simulink model "three_way_newest_1"  (R2025b)
settings: Solver=VariableStepAuto  StartTime=0.0  StopTime=20  RelTol=1e-3
undefined symbols (not defined in the file or in its folder): c, dspblkCoreblockFVToolHelper, gcbh, sfvc784, xck26
libraries: hdlBasic x131, hdlDSPIP x11, simulink x10, hdlUtilities x4, vmcUtilities x1
(part 1 of 2)
settings Model: Creator=janek  LastModifiedBy=janek

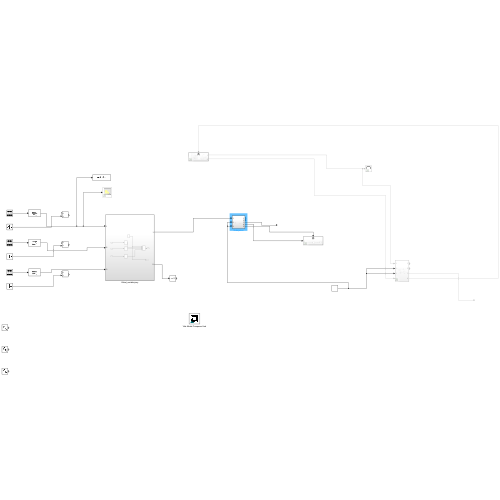
[thumbnail: Simulink's stored preview of the top-level diagram]
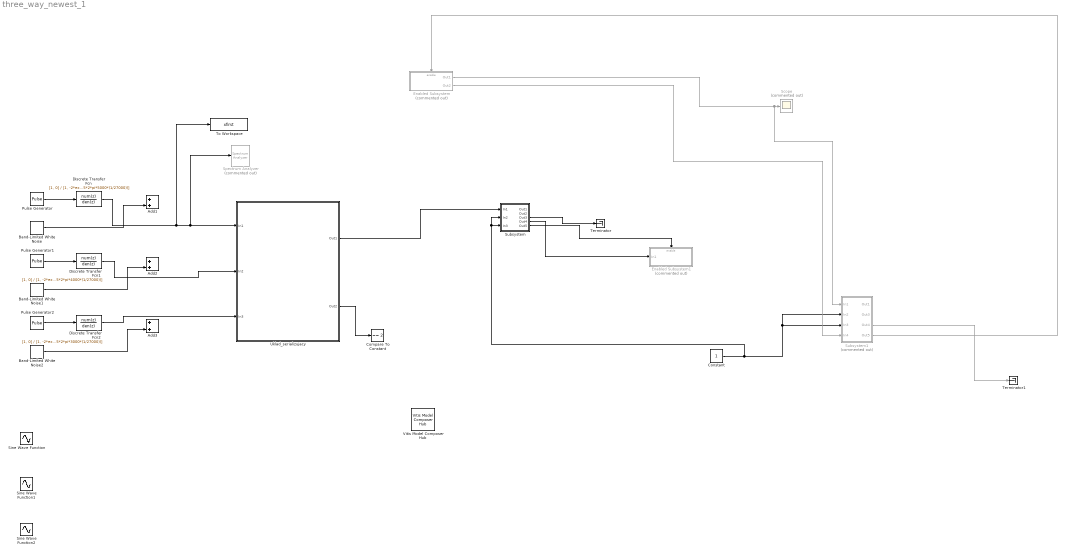
== system three_way_newest_1 ==
  Add1 : Sum
  Add2 : Sum
  Add3 : Sum
  Band-Limited White Noise : simulink/Sources/Band-Limited White Noise  Cov=[0.000001]  Ts=1/27000  seed=[23341]
  Band-Limited White Noise1 : simulink/Sources/Band-Limited White Noise  Cov=[0.000005]  Ts=1/27000  seed=[23341]
  Band-Limited White Noise2 : simulink/Sources/Band-Limited White Noise  Cov=[0.000005]  Ts=1/27000  seed=[23341]
  Compare To Constant : simulink/Logic and Bit Operations/Compare To Constant  relop===  const=2  OutDataTypeStr=boolean
  Constant : Constant
  Discrete Transfer Fcn : DiscreteTransferFcn  LoadFcn=dspblkCoreblockFVToolHelper(gcbh,'load');  Numerator=[1, 0]  Denominator=[1, -2*exp(-0.05*2*pi*5000*(1/27000))*cos(2*pi*5000*sqrt(1-0.05^2)*(1/27000)), exp(-2*0.05*2*pi*5000*(1/27000))]
      settings: CopyFcn=dspblkCoreblockFVToolHelper(gcbh,'copy');  DeleteFcn=dspblkCoreblockFVToolHelper(gcbh,'close');  ModelCloseFcn=dspblkCoreblockFVToolHelper(gcbh,'close');  PreSaveFcn=dspblkCoreblockFVToolHelper(gcbh,'presave');  PostSaveFcn=dspblkCoreblockFVToolHelper(gcbh,'postsave');  CloseFcn=dspblkCoreblockFVToolHelper(gcbh,'close');
  Discrete Transfer Fcn1 : DiscreteTransferFcn  LoadFcn=dspblkCoreblockFVToolHelper(gcbh,'load');  Numerator=[1, 0]  Denominator=[1, -2*exp(-0.05*2*pi*5000*(1/27000))*cos(2*pi*4000*sqrt(1-0.05^2)*(1/27000)), exp(-2*0.05*2*pi*4000*(1/27000))]
      settings: CopyFcn=dspblkCoreblockFVToolHelper(gcbh,'copy');  DeleteFcn=dspblkCoreblockFVToolHelper(gcbh,'close');  ModelCloseFcn=dspblkCoreblockFVToolHelper(gcbh,'close');  PreSaveFcn=dspblkCoreblockFVToolHelper(gcbh,'presave');  PostSaveFcn=dspblkCoreblockFVToolHelper(gcbh,'postsave');  CloseFcn=dspblkCoreblockFVToolHelper(gcbh,'close');
  Discrete Transfer Fcn2 : DiscreteTransferFcn  LoadFcn=dspblkCoreblockFVToolHelper(gcbh,'load');  Numerator=[1, 0]  Denominator=[1, -2*exp(-0.05*2*pi*5000*(1/27000))*cos(2*pi*3000*sqrt(1-0.05^2)*(1/27000)), exp(-2*0.05*2*pi*3000*(1/27000))]
      settings: CopyFcn=dspblkCoreblockFVToolHelper(gcbh,'copy');  DeleteFcn=dspblkCoreblockFVToolHelper(gcbh,'close');  ModelCloseFcn=dspblkCoreblockFVToolHelper(gcbh,'close');  PreSaveFcn=dspblkCoreblockFVToolHelper(gcbh,'presave');  PostSaveFcn=dspblkCoreblockFVToolHelper(gcbh,'postsave');  CloseFcn=dspblkCoreblockFVToolHelper(gcbh,'close');
  Enabled Subsystem : Subsystem  Commented=on  TreatAsAtomicUnit=on
  Enabled Subsystem1 : Subsystem  Commented=on  TreatAsAtomicUnit=on
  Pulse Generator : DiscretePulseGenerator  Period=540  SampleTime=1/27000
  Pulse Generator1 : DiscretePulseGenerator  Period=675  SampleTime=1/27000
  Pulse Generator2 : DiscretePulseGenerator  Period=900  SampleTime=1/27000
  Scope : Scope  Commented=on
      settings: ActiveDisplayYMinimum=-1.152524294390888  ActiveDisplayYMaximum=1.239169366043442  DataLoggingVariableName=ScopeData15
  Sine Wave Function : Sin  Frequency=2*pi*4000  SampleTime=1/27000
  Sine Wave Function1 : Sin  Frequency=2*pi*5000  SampleTime=1/27000
  Sine Wave Function2 : Sin  Frequency=2*pi*3000  SampleTime=1/27000
  Spectrum Analyzer : SpectrumAnalyzer  Commented=on  WindowPosition=[993.000000,73.000000,800.000000,500.000000,]  ScopeFrameLocation=window  WindowInvariantSamplesPerUpdate=on  Span=27000  StartFrequency=-13500  StopFrequency=13500  YLimits=[-53.93 -0.0586]  SelectedToolstripTab=spectrumAnalyzerToolstrip.measurementsTab
  Subsystem : Subsystem
  Subsystem1 : Subsystem  Commented=on
  Terminator : Terminator
  Terminator1 : Terminator
  To Workspace : ToWorkspace  VariableName=xfirst  SampleTime=-1
  Uklad_serializujacy : Subsystem
  Vitis Model Composer Hub : vmcUtilities/Vitis Model Composer Hub  Tag=genX  CodeGeneration=off  SubsystemName=Subsystem  CompilationType=HDLCompilation  ExportTypeV2=IP Catalog  StartColumn=1  NumberOfColumns=1  TargetDirectory=./netlist  exportDesign=off  analyzeDesign=off  validateDesignOnHw=off  ExportType=AI Engines  IpVendor=xilinx.com  IpLibrary=hls  IpVersion=1.0  IpHWLanguage=Verilog  AieCompilerOptions={}  AieSimulatorOptions={}  CreateTestbench=off  TestbenchStackSize=10  RunRtlSim=off  RunCSim=off  RunAieSim=off  AieSimTimeout=50000  RunAieSimProfiling=off  LaunchVitisAnalyzer=off  PlotOutput=off  RunX86Sim=off  X86SimTimeout=10  GenHwImage=off  GenLibadfXo=on  GenHwValidationCode=off  PlatformType=Not Specified  HwSystemType=Baremetal  HwValidationTarget=hw  ProjDevice=Kria KR260 Robotics Starter Kit SOM (xck26-sfvc784-2LV-c)  ProjDevicePart=xck26-sfvc784-2LV-c  AIEType=None  SamplePeriod=-1  ClockFrequency=200  DataPathParallelism=1  xilinxfamily=zynquplus  part=xck26  speed=-2LV-c  package=sfvc784  directory=./netlist\ip\Subsystem\src  testbench=off  incr_netlist=off  synthesis_tool=Vivado  clock_wrapper=Clock Enables  dbl_ovrd=According to Block Masks  dcm_input_clock_period=10  sysclk_period=1000  simulink_period=1/81000  eval_field=0  LogFileName=''  NThreads=4
  wires:
  Discrete Transfer Fcn/1 -> To Workspace/1, Spectrum Analyzer/1, Uklad_serializujacy/1(In1)
  Band-Limited White Noise/1 -> Add1/2
  Discrete Transfer Fcn1/1 -> Uklad_serializujacy/2(In2)
  Pulse Generator1/1 -> Discrete Transfer Fcn1/1
  Band-Limited White Noise1/1 -> Add2/2
  Discrete Transfer Fcn2/1 -> Uklad_serializujacy/3(In3)
  Subsystem1/3(Out4) -> Terminator1/1
  Pulse Generator/1 -> Discrete Transfer Fcn/1
  Constant/1 -> Subsystem/3(In3), Subsystem/2(In2), Subsystem1/2(In2), Subsystem1/3(In3)
  Band-Limited White Noise2/1 -> Add3/2
  Pulse Generator2/1 -> Discrete Transfer Fcn2/1
  Uklad_serializujacy/2(Out2) -> Compare To Constant/1
  Enabled Subsystem/2(Out2) -> Subsystem1/4(In4)
  Enabled Subsystem/1(Out1) -> Scope/1, Subsystem1/1(In1)
  Subsystem1/4(Out5) -> Enabled Subsystem/Enable
  Subsystem/3(Out3) -> Terminator/1
  Uklad_serializujacy/1(Out1) -> Subsystem/1(In1)
  Subsystem/4(Out4) -> Enabled Subsystem1/1(In1)
  Subsystem/5(Out5) -> Enabled Subsystem1/Enable

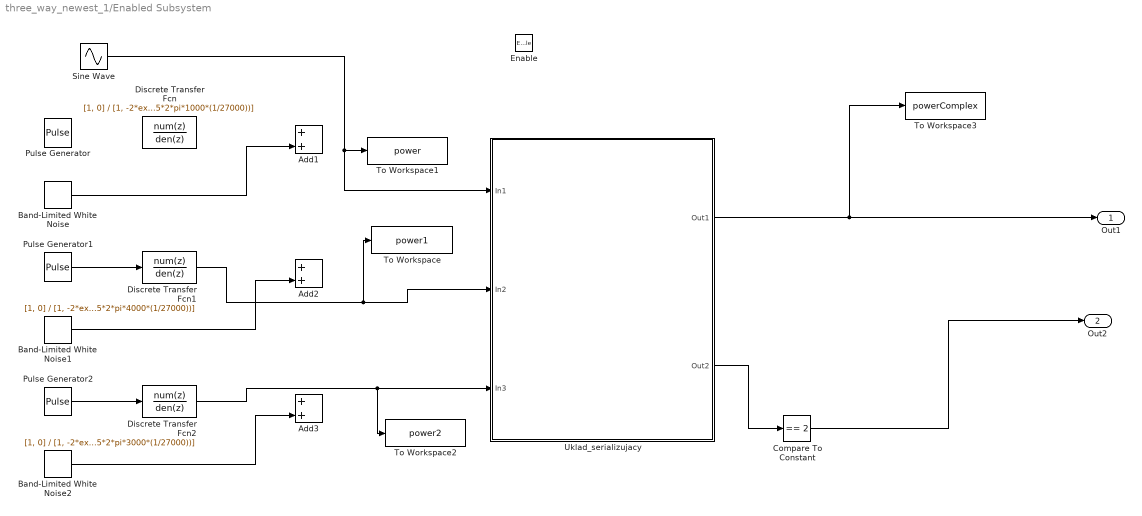
== system three_way_newest_1/Enabled Subsystem ==
  Enable : EnablePort
  Add1 : Sum
  Add2 : Sum
  Add3 : Sum
  Band-Limited White Noise : simulink/Sources/Band-Limited White Noise  Cov=[0.000001]  Ts=1/27000  seed=[23341]
  Band-Limited White Noise1 : simulink/Sources/Band-Limited White Noise  Cov=[0.000005]  Ts=1/27000  seed=[23341]
  Band-Limited White Noise2 : simulink/Sources/Band-Limited White Noise  Cov=[0.000005]  Ts=1/27000  seed=[23341]
  Compare To Constant : simulink/Logic and Bit Operations/Compare To Constant  relop===  const=2  OutDataTypeStr=boolean
  Discrete Transfer Fcn : DiscreteTransferFcn  LoadFcn=dspblkCoreblockFVToolHelper(gcbh,'load');  Numerator=[1, 0]  Denominator=[1, -2*exp(-0.05*2*pi*5000*(1/27000))*cos(2*pi*1000*sqrt(1-0.05^2)*(1/27000)), exp(-2*0.05*2*pi*1000*(1/27000))]
      settings: CopyFcn=dspblkCoreblockFVToolHelper(gcbh,'copy');  DeleteFcn=dspblkCoreblockFVToolHelper(gcbh,'close');  ModelCloseFcn=dspblkCoreblockFVToolHelper(gcbh,'close');  PreSaveFcn=dspblkCoreblockFVToolHelper(gcbh,'presave');  PostSaveFcn=dspblkCoreblockFVToolHelper(gcbh,'postsave');  CloseFcn=dspblkCoreblockFVToolHelper(gcbh,'close');
  Discrete Transfer Fcn1 : DiscreteTransferFcn  LoadFcn=dspblkCoreblockFVToolHelper(gcbh,'load');  Numerator=[1, 0]  Denominator=[1, -2*exp(-0.05*2*pi*5000*(1/27000))*cos(2*pi*4000*sqrt(1-0.05^2)*(1/27000)), exp(-2*0.05*2*pi*4000*(1/27000))]
      settings: CopyFcn=dspblkCoreblockFVToolHelper(gcbh,'copy');  DeleteFcn=dspblkCoreblockFVToolHelper(gcbh,'close');  ModelCloseFcn=dspblkCoreblockFVToolHelper(gcbh,'close');  PreSaveFcn=dspblkCoreblockFVToolHelper(gcbh,'presave');  PostSaveFcn=dspblkCoreblockFVToolHelper(gcbh,'postsave');  CloseFcn=dspblkCoreblockFVToolHelper(gcbh,'close');
  Discrete Transfer Fcn2 : DiscreteTransferFcn  LoadFcn=dspblkCoreblockFVToolHelper(gcbh,'load');  Numerator=[1, 0]  Denominator=[1, -2*exp(-0.05*2*pi*5000*(1/27000))*cos(2*pi*3000*sqrt(1-0.05^2)*(1/27000)), exp(-2*0.05*2*pi*3000*(1/27000))]
      settings: CopyFcn=dspblkCoreblockFVToolHelper(gcbh,'copy');  DeleteFcn=dspblkCoreblockFVToolHelper(gcbh,'close');  ModelCloseFcn=dspblkCoreblockFVToolHelper(gcbh,'close');  PreSaveFcn=dspblkCoreblockFVToolHelper(gcbh,'presave');  PostSaveFcn=dspblkCoreblockFVToolHelper(gcbh,'postsave');  CloseFcn=dspblkCoreblockFVToolHelper(gcbh,'close');
  Pulse Generator : DiscretePulseGenerator  Period=540  SampleTime=1/27000
  Pulse Generator1 : DiscretePulseGenerator  Period=675  SampleTime=1/27000
  Pulse Generator2 : DiscretePulseGenerator  Period=900  SampleTime=1/27000
  Sine Wave : Sin  Frequency=2*pi*1000  SampleTime=1/27000
  To Workspace : ToWorkspace  VariableName=power1  SampleTime=-1
  To Workspace1 : ToWorkspace  VariableName=power  SampleTime=-1
  To Workspace2 : ToWorkspace  VariableName=power2  SampleTime=-1
  To Workspace3 : ToWorkspace  VariableName=powerComplex  SampleTime=-1
  Uklad_serializujacy : Subsystem
  Out1 : Outport
  Out2 : Outport  Port=2
  wires:
  Band-Limited White Noise/1 -> Add1/2
  Pulse Generator2/1 -> Discrete Transfer Fcn2/1
  Discrete Transfer Fcn1/1 -> To Workspace/1, Uklad_serializujacy/2(In2)
  Discrete Transfer Fcn2/1 -> To Workspace2/1, Uklad_serializujacy/3(In3)
  Band-Limited White Noise1/1 -> Add2/2
  Uklad_serializujacy/2(Out2) -> Compare To Constant/1
  Band-Limited White Noise2/1 -> Add3/2
  Pulse Generator1/1 -> Discrete Transfer Fcn1/1
  Uklad_serializujacy/1(Out1) -> To Workspace3/1, Out1/1
  Compare To Constant/1 -> Out2/1
  Sine Wave/1 -> Uklad_serializujacy/1(In1), To Workspace1/1

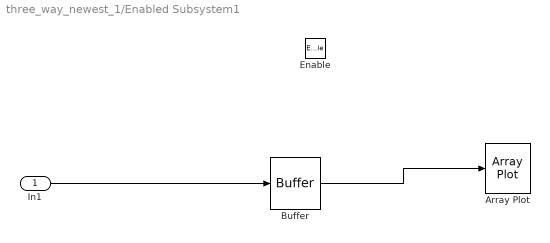
== system three_way_newest_1/Enabled Subsystem1 ==
  In1 : Inport
  Enable : EnablePort
  Array Plot : ArrayPlot  WindowPosition=[372.000000,68.000000,800.000000,500.000000,]  ScopeFrameLocation=window  YLimits=[0.875 1.125]
  Buffer : Buffer  N=4096  OutputFrames=off
  wires:
  In1/1 -> Buffer/1
  Buffer/1 -> Array Plot/1

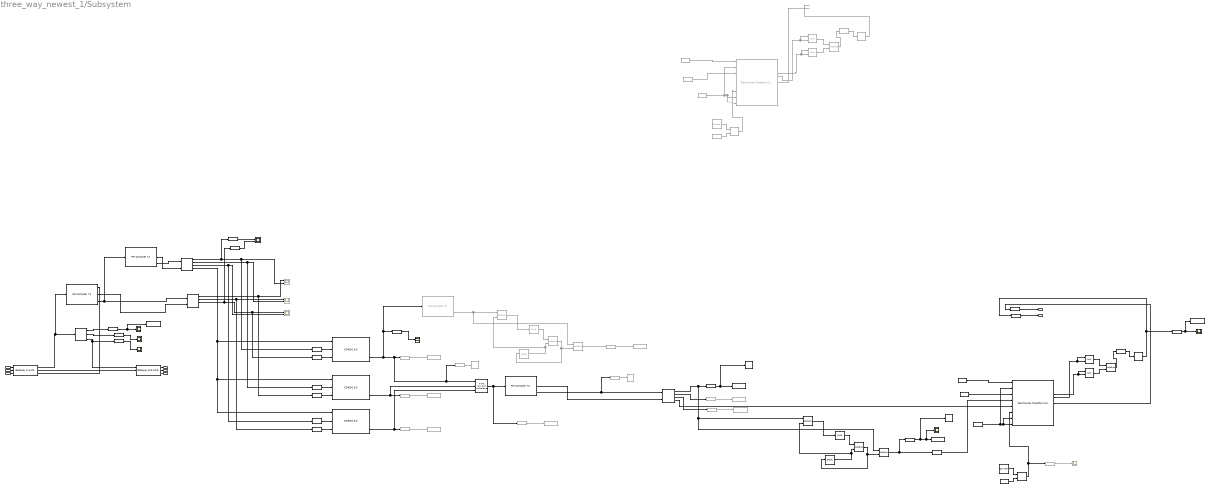
== system three_way_newest_1/Subsystem ==
  In1 : Inport
  In2 : Inport  Port=2
  In3 : Inport  Port=3
  AddSub : hdlBasic/AddSub  Commented=on  mode=Addition  use_carryin=off  use_carryout=off  en=off  latency=0  precision=User Defined  arith_type="Signed  (2's comp)"  n_bits=32  bin_pt=26  quantization="Round  (unbiased: +/- Inf)"  overflow=Wrap  use_behavioral_HDL=off  hw_selection=Fabric  pipelined=off  XmcBlockStatus=1  maskContainerNames=tabcontainer1  block_type=addsub  block_config=sysgen:Addsub_config
  AddSub1 : hdlBasic/AddSub  Commented=on  mode=Subtraction  use_carryin=off  use_carryout=off  en=off  latency=0  precision=User Defined  arith_type="Signed  (2's comp)"  n_bits=32  bin_pt=26  quantization="Round  (unbiased: +/- Inf)"  overflow=Wrap  use_behavioral_HDL=off  hw_selection=Fabric  pipelined=off  XmcBlockStatus=1  maskContainerNames=tabcontainer1  block_type=addsub  block_config=sysgen:Addsub_config
  AddSub2 : hdlBasic/AddSub  Commented=on  mode=Subtraction  use_carryin=off  use_carryout=off  en=off  latency=0  precision=User Defined  arith_type="Signed  (2's comp)"  n_bits=16  bin_pt=12  quantization="Round  (unbiased: +/- Inf)"  overflow=Saturate  use_behavioral_HDL=off  hw_selection=Fabric  pipelined=off  XmcBlockStatus=1  maskContainerNames=tabcontainer1  block_type=addsub  block_config=sysgen:Addsub_config
  AddSub3 : hdlBasic/AddSub  mode=Addition  use_carryin=off  use_carryout=off  en=off  latency=0  precision=Full  arith_type=Unsigned  n_bits=16  bin_pt=14  quantization=Truncate  overflow=Wrap  use_behavioral_HDL=off  hw_selection=Fabric  pipelined=off  XmcBlockStatus=1  maskContainerNames=tabcontainer1  block_type=addsub  block_config=sysgen:Addsub_config
  AddSub4 : hdlBasic/AddSub  Commented=on  mode=Addition  use_carryin=off  use_carryout=off  en=off  latency=0  precision=Full  arith_type=Unsigned  n_bits=16  bin_pt=14  quantization=Truncate  overflow=Wrap  use_behavioral_HDL=off  hw_selection=Fabric  pipelined=off  XmcBlockStatus=1  maskContainerNames=tabcontainer1  block_type=addsub  block_config=sysgen:Addsub_config
  AddSub5 : hdlBasic/AddSub  mode=Addition  use_carryin=off  use_carryout=off  en=off  latency=0  precision=User Defined  arith_type="Signed  (2's comp)"  n_bits=32  bin_pt=26  quantization="Round  (unbiased: +/- Inf)"  overflow=Wrap  use_behavioral_HDL=off  hw_selection=Fabric  pipelined=off  XmcBlockStatus=1  maskContainerNames=tabcontainer1  block_type=addsub  block_config=sysgen:Addsub_config
  AddSub6 : hdlBasic/AddSub  mode=Subtraction  use_carryin=off  use_carryout=off  en=off  latency=0  precision=User Defined  arith_type="Signed  (2's comp)"  n_bits=32  bin_pt=26  quantization="Round  (unbiased: +/- Inf)"  overflow=Wrap  use_behavioral_HDL=off  hw_selection=Fabric  pipelined=off  XmcBlockStatus=1  maskContainerNames=tabcontainer1  block_type=addsub  block_config=sysgen:Addsub_config
  AddSub7 : hdlBasic/AddSub  mode=Subtraction  use_carryin=off  use_carryout=off  en=off  latency=0  precision=User Defined  arith_type="Signed  (2's comp)"  n_bits=16  bin_pt=12  quantization="Round  (unbiased: +/- Inf)"  overflow=Saturate  use_behavioral_HDL=off  hw_selection=Fabric  pipelined=off  XmcBlockStatus=1  maskContainerNames=tabcontainer1  block_type=addsub  block_config=sysgen:Addsub_config
  "CORDIC 6.0 " : hdlDSPIP/CORDIC 6.0   functional_selection=Translate  architectural_configuration=Parallel  pipelining_mode=Maximum  data_format=SignedFraction  phase_format=Radians  input_width=16  output_width=16  round_mode=Nearest_Even  iterations=0  precision=0  compensation_scaling=BRAM  coarse_rotation=on  aclken=off  aresetn=off  out_tready=off  cartesian_has_tuser=off  cartesian_has_tlast=off  cartesian_tuser_width=1  phase_has_tuser=off  phase_has_tlast=off  phase_tuser_width=1  out_tlast_behv=Null  flow_control=NonBlocking  optimize_goal=Resources  trim_axipin_name=on  simulation_type=hybrid_sim  simulation_model=sysgen:cordic_v6_0  data_path_portlist={'s_axis_cartesian_tdata_imag', 's_axis_cartesian_tdata_real', 's_axis_phase_tdata_phase', 'm_axis_dout_tdata_imag', 'm_axis_dout_tdata_real', 'm_axis_dout_tdata_phase','m_axis_dout_tdata'}  ip_name=CORDIC  ip_version=6.0  dsptool_ready=true  ipcore_usecache=true  ipcore_useipmodelcache=true  wrapper_available=true  port_translation_map={ 'aclken' => 'en', 'aresetn' => 'rst' }  XmcBlockStatus=1  maskContainerNames=group15  block_type=cordic_v6_0  block_config=sysgen:rodinimport_config  block_width=800
  CORDIC 6.0 1 : hdlDSPIP/CORDIC 6.0   functional_selection=Translate  architectural_configuration=Parallel  pipelining_mode=Maximum  data_format=SignedFraction  phase_format=Radians  input_width=16  output_width=16  round_mode=Nearest_Even  iterations=0  precision=0  compensation_scaling=BRAM  coarse_rotation=on  aclken=off  aresetn=off  out_tready=off  cartesian_has_tuser=off  cartesian_has_tlast=off  cartesian_tuser_width=1  phase_has_tuser=off  phase_has_tlast=off  phase_tuser_width=1  out_tlast_behv=Null  flow_control=NonBlocking  optimize_goal=Resources  trim_axipin_name=on  simulation_type=hybrid_sim  simulation_model=sysgen:cordic_v6_0  data_path_portlist={'s_axis_cartesian_tdata_imag', 's_axis_cartesian_tdata_real', 's_axis_phase_tdata_phase', 'm_axis_dout_tdata_imag', 'm_axis_dout_tdata_real', 'm_axis_dout_tdata_phase','m_axis_dout_tdata'}  ip_name=CORDIC  ip_version=6.0  dsptool_ready=true  ipcore_usecache=true  ipcore_useipmodelcache=true  wrapper_available=true  port_translation_map={ 'aclken' => 'en', 'aresetn' => 'rst' }  XmcBlockStatus=1  maskContainerNames=group15  block_type=cordic_v6_0  block_config=sysgen:rodinimport_config  block_width=800
  CORDIC 6.0 2 : hdlDSPIP/CORDIC 6.0   functional_selection=Translate  architectural_configuration=Parallel  pipelining_mode=Maximum  data_format=SignedFraction  phase_format=Radians  input_width=16  output_width=16  round_mode=Nearest_Even  iterations=0  precision=0  compensation_scaling=BRAM  coarse_rotation=on  aclken=off  aresetn=off  out_tready=off  cartesian_has_tuser=off  cartesian_has_tlast=off  cartesian_tuser_width=1  phase_has_tuser=off  phase_has_tlast=off  phase_tuser_width=1  out_tlast_behv=Null  flow_control=NonBlocking  optimize_goal=Resources  trim_axipin_name=on  simulation_type=hybrid_sim  simulation_model=sysgen:cordic_v6_0  data_path_portlist={'s_axis_cartesian_tdata_imag', 's_axis_cartesian_tdata_real', 's_axis_phase_tdata_phase', 'm_axis_dout_tdata_imag', 'm_axis_dout_tdata_real', 'm_axis_dout_tdata_phase','m_axis_dout_tdata'}  ip_name=CORDIC  ip_version=6.0  dsptool_ready=true  ipcore_usecache=true  ipcore_useipmodelcache=true  wrapper_available=true  port_translation_map={ 'aclken' => 'en', 'aresetn' => 'rst' }  XmcBlockStatus=1  maskContainerNames=group15  block_type=cordic_v6_0  block_config=sysgen:rodinimport_config  block_width=800
  Constant : hdlBasic/Constant  Commented=on  const=0  gui_display_data_type=Fixed-point  arith_type=Signed (2's comp)  n_bits=16  bin_pt=15  preci_type=Single  exp_width=8  frac_width=24  explicit_period=off  period=1  XmcBlockStatus=1  maskContainerNames=tabcontainer1  block_type=constant  block_config=sysgen:Constant_config
  Constant1 : hdlBasic/Constant  Commented=on  const=1  gui_display_data_type=Boolean  arith_type=Boolean  n_bits=1  bin_pt=0  preci_type=Single  exp_width=8  frac_width=24  explicit_period=off  period=1  XmcBlockStatus=1  maskContainerNames=tabcontainer1  block_type=constant  block_config=sysgen:Constant_config
  Constant2 : hdlBasic/Constant  const=0  gui_display_data_type=Fixed-point  arith_type=Signed (2's comp)  n_bits=16  bin_pt=15  preci_type=Single  exp_width=8  frac_width=24  explicit_period=off  period=1  XmcBlockStatus=1  maskContainerNames=tabcontainer1  block_type=constant  block_config=sysgen:Constant_config
  Constant3 : hdlBasic/Constant  Commented=on  const=1  gui_display_data_type=Fixed-point  arith_type=Unsigned  n_bits=1  bin_pt=0  preci_type=Single  exp_width=8  frac_width=24  explicit_period=off  period=1  XmcBlockStatus=1  maskContainerNames=tabcontainer1  block_type=constant  block_config=sysgen:Constant_config
  Constant4 : hdlBasic/Constant  Commented=on  const=4095  gui_display_data_type=Fixed-point  arith_type=Unsigned  n_bits=12  bin_pt=0  preci_type=Single  exp_width=8  frac_width=24  explicit_period=off  period=1  XmcBlockStatus=1  maskContainerNames=tabcontainer1  block_type=constant  block_config=sysgen:Constant_config
  Constant5 : hdlBasic/Constant  const=1  gui_display_data_type=Boolean  arith_type=Boolean  n_bits=1  bin_pt=0  preci_type=Single  exp_width=8  frac_width=24  explicit_period=off  period=1  XmcBlockStatus=1  maskContainerNames=tabcontainer1  block_type=constant  block_config=sysgen:Constant_config
  Constant6 : hdlBasic/Constant  const=1  gui_display_data_type=Fixed-point  arith_type=Unsigned  n_bits=1  bin_pt=0  preci_type=Single  exp_width=8  frac_width=24  explicit_period=off  period=1  XmcBlockStatus=1  maskContainerNames=tabcontainer1  block_type=constant  block_config=sysgen:Constant_config
  Constant7 : hdlBasic/Constant  const=4095  gui_display_data_type=Fixed-point  arith_type=Unsigned  n_bits=12  bin_pt=0  preci_type=Single  exp_width=8  frac_width=24  explicit_period=off  period=1  XmcBlockStatus=1  maskContainerNames=tabcontainer1  block_type=constant  block_config=sysgen:Constant_config
  Convert{1,3..7} (6 alike) : hdlBasic/Convert  gui_display_data_type=Fixed-point  arith_type=Signed (2's comp)  n_bits=16  bin_pt=14  float_type=Single  exp_bits=8  fraction_bits=24  quantization="Round  (unbiased: +/- Inf)"  overflow=Saturate  en=off  latency=0  pipeline=off  XmcBlockStatus=1  maskContainerNames=group2  block_type=convert  block_config=sysgen:Convert_config  block_width=595  block_height=885
  Convert2 : hdlBasic/Convert  Commented=on  gui_display_data_type=Floating-point  arith_type=Floating-point  n_bits=16  bin_pt=14  float_type=Single  exp_bits=8  fraction_bits=24  quantization="Round  (unbiased: +/- Inf)"  overflow=Saturate  en=off  latency=0  pipeline=off  XmcBlockStatus=1  maskContainerNames=group2  block_type=convert  block_config=sysgen:Convert_config  block_width=595  block_height=885
  Convert8 : hdlBasic/Convert  gui_display_data_type=Floating-point  arith_type=Floating-point  n_bits=16  bin_pt=14  float_type=Single  exp_bits=8  fraction_bits=24  quantization="Round  (unbiased: +/- Inf)"  overflow=Saturate  en=off  latency=0  pipeline=off  XmcBlockStatus=1  maskContainerNames=group2  block_type=convert  block_config=sysgen:Convert_config  block_width=595  block_height=885
  Convert9 : hdlBasic/Convert  gui_display_data_type=Fixed-point  arith_type=Signed (2's comp)  n_bits=16  bin_pt=15  float_type=Single  exp_bits=8  fraction_bits=24  quantization="Round  (unbiased: +/- Inf)"  overflow=Saturate  en=off  latency=0  pipeline=off  XmcBlockStatus=1  maskContainerNames=group2  block_type=convert  block_config=sysgen:Convert_config  block_width=595  block_height=885
  Counter : hdlBasic/Counter  Commented=on  cnt_type=Count limited  cnt_to=4095  operation=Up  start_count=0  cnt_by_val=1  arith_type=Unsigned  n_bits=12  bin_pt=0  load_pin=off  rst=off  en=off  explicit_period=Explicit  period=1  use_behavioral_HDL=off  implementation=Fabric  XmcBlockStatus=1  maskContainerNames=group1  block_type=counter  block_config=sysgen:Counter_config  block_width=531  block_height=1023
  Counter1 : hdlBasic/Counter  cnt_type=Count limited  cnt_to=4095  operation=Up  start_count=0  cnt_by_val=1  arith_type=Unsigned  n_bits=12  bin_pt=0  load_pin=off  rst=off  en=off  explicit_period=Explicit  period=1  use_behavioral_HDL=off  implementation=Fabric  XmcBlockStatus=1  maskContainerNames=group1  block_type=counter  block_config=sysgen:Counter_config  block_width=531  block_height=1023
  Delay1 : hdlBasic/Delay  Commented=on  rst=off  en=off  latency=1  reg_retiming=off  XmcBlockStatus=1  maskContainerNames=group1  block_type=delay  block_config=sysgen:Delay_config
  Delay2 : hdlBasic/Delay  rst=off  en=off  latency=1  reg_retiming=off  XmcBlockStatus=1  maskContainerNames=group1  block_type=delay  block_config=sysgen:Delay_config
  "FIR Compiler 7.2 " : hdlDSPIP/FIR Compiler 7.2   coefficientvector=my_coefficients  coefficient_sets=1  coefficient_reload=off  filter_type=Single_Rate  rate_change_type=Integer  interpolation_rate=1  decimation_rate=1  zero_pack_factor=1  channel_sequence=Basic  number_channels=3  pattern_list='P4-0,P4-1,P4-2,P4-3,P4-4'  number_paths=1  ratespecification=Maximum_Possible  sampleperiod=1  hardwareoversamplingrate=1  coefficient_sign=Unsigned  quantization=Quantize_Only  coefficient_width=16  bestprecision=on  coefficient_fractional_bits=8  coefficient_structure=Inferred  output_rounding_mode=Convergent_Rounding_to_Even  output_width=16  filter_architecture=Systolic_Multiply_Accumulate  optimization_goal=Area  optimization_list='None'  data_buffer_type=Automatic  coefficient_buffer_type=Automatic  input_buffer_type=Automatic  output_buffer_type=Automatic  preference_for_other_storage=Automatic  multi_column_support=Automatic  columnconfig='11'  inter_column_pipe_length=4  data_has_tlast=Not_Required  m_data_has_tready=off  s_data_has_fifo=off  s_data_has_tuser=Not_Required  m_data_has_tuser=Not_Required  s_config_sync_mode=On_Vector  s_config_method=Single  num_reload_slots=1  has_aclken=off  has_aresetn=off  reset_data_vector=on  trim_axipin_name=on  simulation_type=hybrid_sim  simulation_model=sysgen:xfirv7_2_cmodel  data_path_portlist={ 's_axis_data_tdata', 'm_axis_data_tdata' }  passband_min=0.0  passband_max=0.5  stopband_min=0.5  stopband_max=1.0  filter_selection=1  gui_behaviour='Sysgen_GUI'  data_sign=Signed  data_width=16  data_fractional_bits=0  data_tuser_width=1  wrapper_available=true  ip_wrap_arbitrary_binary_point=true  ip_name=FIR Compiler  ip_version=7.2  dsptool_ready=true  ipcore_usecache=true  ipcore_useipmodelcache=true  port_translation_map={ 'aclken' => 'en', 'aresetn' => 'rst' }  run_core_at_system_period=true  ipcore_xco_need_fpga_part=true  ipcore_fpga_part=[]  XmcBlockStatus=1  maskContainerNames=tabcontainer1  block_type=fir_compiler_v7_2  block_config=sysgen:rodinimport_config  block_width=820  block_height=600
  FIR Compiler 7.2 1 : hdlDSPIP/FIR Compiler 7.2   coefficientvector=hilbert  coefficient_sets=1  coefficient_reload=off  filter_type=Single_Rate  rate_change_type=Integer  interpolation_rate=1  decimation_rate=1  zero_pack_factor=1  channel_sequence=Basic  number_channels=3  pattern_list='P4-0,P4-1,P4-2,P4-3,P4-4'  number_paths=1  ratespecification=Maximum_Possible  sampleperiod=1  hardwareoversamplingrate=1  coefficient_sign=Unsigned  quantization=Quantize_Only  coefficient_width=16  bestprecision=on  coefficient_fractional_bits=8  coefficient_structure=Inferred  output_rounding_mode=Convergent_Rounding_to_Even  output_width=16  filter_architecture=Systolic_Multiply_Accumulate  optimization_goal=Area  optimization_list='None'  data_buffer_type=Automatic  coefficient_buffer_type=Automatic  input_buffer_type=Automatic  output_buffer_type=Automatic  preference_for_other_storage=Automatic  multi_column_support=Automatic  columnconfig='11'  inter_column_pipe_length=4  data_has_tlast=Not_Required  m_data_has_tready=off  s_data_has_fifo=off  s_data_has_tuser=Not_Required  m_data_has_tuser=Not_Required  s_config_sync_mode=On_Vector  s_config_method=Single  num_reload_slots=1  has_aclken=off  has_aresetn=off  reset_data_vector=on  trim_axipin_name=on  simulation_type=hybrid_sim  simulation_model=sysgen:xfirv7_2_cmodel  data_path_portlist={ 's_axis_data_tdata', 'm_axis_data_tdata' }  passband_min=0.0  passband_max=0.5  stopband_min=0.5  stopband_max=1.0  filter_selection=1  gui_behaviour='Sysgen_GUI'  data_sign=Signed  data_width=16  data_fractional_bits=0  data_tuser_width=1  wrapper_available=true  ip_wrap_arbitrary_binary_point=true  ip_name=FIR Compiler  ip_version=7.2  dsptool_ready=true  ipcore_usecache=true  ipcore_useipmodelcache=true  port_translation_map={ 'aclken' => 'en', 'aresetn' => 'rst' }  run_core_at_system_period=true  ipcore_xco_need_fpga_part=true  ipcore_fpga_part=[]  XmcBlockStatus=1  maskContainerNames=tabcontainer1  block_type=fir_compiler_v7_2  block_config=sysgen:rodinimport_config  block_width=820  block_height=600
  FIR Compiler 7.2 2 : hdlDSPIP/FIR Compiler 7.2   Commented=on  coefficientvector=[6,0,-4,-3,5,6,-6,-13,7,44,64,44,7,-13,-6,6,5,-3,-4,0,6]  coefficient_sets=1  coefficient_reload=off  filter_type=Single_Rate  rate_change_type=Integer  interpolation_rate=1  decimation_rate=1  zero_pack_factor=1  channel_sequence=Basic  number_channels=1  pattern_list='P4-0,P4-1,P4-2,P4-3,P4-4'  number_paths=1  ratespecification=Maximum_Possible  sampleperiod=1  hardwareoversamplingrate=1  coefficient_sign=Signed  quantization=Integer_Coefficients  coefficient_width=16  bestprecision=off  coefficient_fractional_bits=0  coefficient_structure=Inferred  output_rounding_mode=Full_Precision  output_width=24  filter_architecture=Systolic_Multiply_Accumulate  optimization_goal=Area  optimization_list='None'  data_buffer_type=Automatic  coefficient_buffer_type=Automatic  input_buffer_type=Automatic  output_buffer_type=Automatic  preference_for_other_storage=Automatic  multi_column_support=Automatic  columnconfig='11'  inter_column_pipe_length=4  data_has_tlast=Not_Required  m_data_has_tready=off  s_data_has_fifo=off  s_data_has_tuser=Not_Required  m_data_has_tuser=Not_Required  s_config_sync_mode=On_Vector  s_config_method=Single  num_reload_slots=1  has_aclken=off  has_aresetn=off  reset_data_vector=on  trim_axipin_name=on  simulation_type=hybrid_sim  simulation_model=sysgen:xfirv7_2_cmodel  data_path_portlist={ 's_axis_data_tdata', 'm_axis_data_tdata' }  passband_min=0.0  passband_max=0.5  stopband_min=0.5  stopband_max=1.0  filter_selection=1  gui_behaviour='Sysgen_GUI'  data_sign=Signed  data_width=16  data_fractional_bits=0  data_tuser_width=1  wrapper_available=true  ip_wrap_arbitrary_binary_point=true  ip_name=FIR Compiler  ip_version=7.2  dsptool_ready=true  ipcore_usecache=true  ipcore_useipmodelcache=true  port_translation_map={ 'aclken' => 'en', 'aresetn' => 'rst' }  run_core_at_system_period=true  ipcore_xco_need_fpga_part=true  ipcore_fpga_part=[]  XmcBlockStatus=1  maskContainerNames=tabcontainer1  block_type=fir_compiler_v7_2  block_config=sysgen:rodinimport_config  block_width=820  block_height=600
  FIR Compiler 7.2 3 : hdlDSPIP/FIR Compiler 7.2   coefficientvector=decimation_fir  coefficient_sets=1  coefficient_reload=off  filter_type=Decimation  rate_change_type=Integer  interpolation_rate=1  decimation_rate=10  zero_pack_factor=1  channel_sequence=Basic  number_channels=3  pattern_list='P4-0,P4-1,P4-2,P4-3,P4-4'  number_paths=1  ratespecification=Maximum_Possible  sampleperiod=1  hardwareoversamplingrate=1  coefficient_sign=Unsigned  quantization=Quantize_Only  coefficient_width=16  bestprecision=on  coefficient_fractional_bits=8  coefficient_structure=Inferred  output_rounding_mode=Convergent_Rounding_to_Even  output_width=16  filter_architecture=Systolic_Multiply_Accumulate  optimization_goal=Area  optimization_list='None'  data_buffer_type=Automatic  coefficient_buffer_type=Automatic  input_buffer_type=Automatic  output_buffer_type=Automatic  preference_for_other_storage=Automatic  multi_column_support=Automatic  columnconfig='2'  inter_column_pipe_length=4  data_has_tlast=Not_Required  m_data_has_tready=off  s_data_has_fifo=off  s_data_has_tuser=Not_Required  m_data_has_tuser=Not_Required  s_config_sync_mode=On_Vector  s_config_method=Single  num_reload_slots=1  has_aclken=off  has_aresetn=off  reset_data_vector=on  trim_axipin_name=on  simulation_type=hybrid_sim  simulation_model=sysgen:xfirv7_2_cmodel  data_path_portlist={ 's_axis_data_tdata', 'm_axis_data_tdata' }  passband_min=0.0  passband_max=0.5  stopband_min=0.5  stopband_max=1.0  filter_selection=1  gui_behaviour='Sysgen_GUI'  data_sign=Signed  data_width=16  data_fractional_bits=0  data_tuser_width=1  wrapper_available=true  ip_wrap_arbitrary_binary_point=true  ip_name=FIR Compiler  ip_version=7.2  dsptool_ready=true  ipcore_usecache=true  ipcore_useipmodelcache=true  port_translation_map={ 'aclken' => 'en', 'aresetn' => 'rst' }  run_core_at_system_period=true  ipcore_xco_need_fpga_part=true  ipcore_fpga_part=[]  XmcBlockStatus=1  maskContainerNames=tabcontainer1  block_type=fir_compiler_v7_2  block_config=sysgen:rodinimport_config  block_width=820  block_height=600
  "Fast Fourier Transform 9.1 " : hdlDSPIP/Fast Fourier Transform 9.1   Commented=on  transform_length=4096  target_clock_frequency=100  target_data_throughput=50  implementation_options=radix_4_burst_io  run_time_configurable_transform_length=off  enable_ssr=off  super_sample_rates=1  data_format=fixed_point  phase_factor_width=24  scaling_options=block_floating_point  rounding_modes=truncation  aclken=off  aresetn=off  output_ordering=natural_order  cyclic_prefix_insertion=off  throttle_scheme=nonrealtime  xk_index=off  ovflo=off  trim_axipin_name=on  memory_options_data=block_ram  memory_options_phase_factors=block_ram  number_of_stages_using_block_ram_for_data_and_phase_factors=1  memory_options_reorder=block_ram  memory_options_hybrid=off  complex_mult_type=use_mults_resources  butterfly_type=use_luts  simulation_type=hybrid_sim  simulation_model=sysgen:xfftv9_cmodel  data_path_portlist={ 's_axis_data_tdata', 'm_axis_data_tdata', 'm_axis_status_tdata', 'event_fft_overflow' }  channels=1  input_ordering=natural_order  input_width=16  ip_name=Fast Fourier Transform  ip_version=9.1  dsptool_ready=true  ipcore_usecache=true  ipcore_useipmodelcache=true  wrapper_available=true  port_translation_map={ 'aclken' => 'en', 'aresetn' => 'rst'}  XmcBlockStatus=1  maskContainerNames=tabcontainer1  block_type=xfft_v9_1  block_config=sysgen:rodinimport_config
  Fast Fourier Transform 9.1 1 : hdlDSPIP/Fast Fourier Transform 9.1   transform_length=4096  target_clock_frequency=1  target_data_throughput=50  implementation_options=radix_4_burst_io  run_time_configurable_transform_length=off  enable_ssr=off  super_sample_rates=1  data_format=fixed_point  phase_factor_width=24  scaling_options=block_floating_point  rounding_modes=truncation  aclken=off  aresetn=off  output_ordering=natural_order  cyclic_prefix_insertion=off  throttle_scheme=nonrealtime  xk_index=off  ovflo=off  trim_axipin_name=on  memory_options_data=block_ram  memory_options_phase_factors=block_ram  number_of_stages_using_block_ram_for_data_and_phase_factors=1  memory_options_reorder=block_ram  memory_options_hybrid=off  complex_mult_type=use_mults_resources  butterfly_type=use_luts  simulation_type=hybrid_sim  simulation_model=sysgen:xfftv9_cmodel  data_path_portlist={ 's_axis_data_tdata', 'm_axis_data_tdata', 'm_axis_status_tdata', 'event_fft_overflow' }  channels=1  input_ordering=natural_order  input_width=16  ip_name=Fast Fourier Transform  ip_version=9.1  dsptool_ready=true  ipcore_usecache=true  ipcore_useipmodelcache=true  wrapper_available=true  port_translation_map={ 'aclken' => 'en', 'aresetn' => 'rst'}  XmcBlockStatus=1  maskContainerNames=tabcontainer1  block_type=xfft_v9_1  block_config=sysgen:rodinimport_config
  Gateway In AXIS : hdlUtilities/Gateway In AXIS  gui_display_data_type=Fixed-point  arith_type=Signed (2's comp)  n_bits=16  bin_pt=14  preci_type=Custom  exp_width=16  frac_width=24  quantization="Round  (unbiased: +/- Inf)"  overflow=Wrap  bool_to_boolean=off  OutSampleTime=1/81000  block_type=gatewayinaxi  XmcBlockStatus=1
  Gateway Out{,7,10..11,13,15..20} (11 alike) : hdlBasic/Gateway Out  inherit_from_input=off  bool_to_boolean=off  hdl_port=on  rows=1  columns=1  UseAsDAC=off  DACChannel='1'  interface=None  automatic_assignment=on  address_offset=hex2dec('00')  intf_name=''  intf_description=''  timing_constraint=None  locs_specified=off  LOCs={}  io_standard={}  XmcBlockStatus=1  maskContainerNames=group4  block_type=gatewayout  block_config=sysgen:gateway_out_config  block_width_w=590  block_height_w=620  block_width=620  block_height=750
  Gateway Out AXIS : hdlUtilities/Gateway Out AXIS  mask_sample_period=1/81000  bool_to_boolean=off  block_type=gatewayoutaxi
  Gateway Out{1..6,8..9,12,14} (10 alike) : hdlBasic/Gateway Out  Commented=on  inherit_from_input=off  bool_to_boolean=off  hdl_port=on  rows=1  columns=1  UseAsDAC=off  DACChannel='1'  interface=None  automatic_assignment=on  address_offset=hex2dec('00')  intf_name=''  intf_description=''  timing_constraint=None  locs_specified=off  LOCs={}  io_standard={}  XmcBlockStatus=1  maskContainerNames=group4  block_type=gatewayout  block_config=sysgen:gateway_out_config  block_width_w=590  block_height_w=620  block_width=620  block_height=750
  Mult1 : hdlBasic/Mult  precision=User Defined  arith_type="Signed  (2's comp)"  n_bits=16  bin_pt=14  quantization="Round  (unbiased: +/- Inf)"  overflow=Saturate  en=off  latency=0  opt_float=off  fp_mult_usage=No Usage  use_behavioral_HDL=off  opt=Speed  use_embedded=on  optimum_pipeline=off  pipeline=on  use_rpm=on  placement_style=Triangular  XmcBlockStatus=1  maskContainerNames=group1  block_type=mult  block_config=sysgen:Mult_config  block_width=598  block_height=876
  Mult2 : hdlBasic/Mult  Commented=on  precision=User Defined  arith_type="Signed  (2's comp)"  n_bits=16  bin_pt=14  quantization="Round  (unbiased: +/- Inf)"  overflow=Saturate  en=off  latency=0  opt_float=off  fp_mult_usage=No Usage  use_behavioral_HDL=off  opt=Speed  use_embedded=on  optimum_pipeline=off  pipeline=on  use_rpm=on  placement_style=Triangular  XmcBlockStatus=1  maskContainerNames=group1  block_type=mult  block_config=sysgen:Mult_config  block_width=598  block_height=876
  Mult3 : hdlBasic/Mult  Commented=on  precision=User Defined  arith_type="Signed  (2's comp)"  n_bits=16  bin_pt=14  quantization="Round  (unbiased: +/- Inf)"  overflow=Saturate  en=off  latency=0  opt_float=off  fp_mult_usage=No Usage  use_behavioral_HDL=off  opt=Speed  use_embedded=on  optimum_pipeline=off  pipeline=on  use_rpm=on  placement_style=Triangular  XmcBlockStatus=1  maskContainerNames=group1  block_type=mult  block_config=sysgen:Mult_config  block_width=598  block_height=876
  Mult4 : hdlBasic/Mult  precision=User Defined  arith_type="Signed  (2's comp)"  n_bits=16  bin_pt=14  quantization="Round  (unbiased: +/- Inf)"  overflow=Saturate  en=off  latency=0  opt_float=off  fp_mult_usage=No Usage  use_behavioral_HDL=off  opt=Speed  use_embedded=on  optimum_pipeline=off  pipeline=on  use_rpm=on  placement_style=Triangular  XmcBlockStatus=1  maskContainerNames=group1  block_type=mult  block_config=sysgen:Mult_config  block_width=598  block_height=876
  Relational : hdlBasic/Relational  Commented=on  mode=a=b  op_type=Bool  en=off  latency=0  XmcBlockStatus=1  maskContainerNames=tabcontainer1  block_type=relational  block_config=sysgen:Relational_config
  Relational1 : hdlBasic/Relational  mode=a=b  op_type=Bool  en=off  latency=0  XmcBlockStatus=1  maskContainerNames=tabcontainer1  block_type=relational  block_config=sysgen:Relational_config
  Scope : Scope  Commented=on
      settings: DataLoggingVariableName=ScopeData28
  Scope{1..2,6..7} (4 alike) : Scope
      Scope1 settings: ActiveDisplayYMinimum=-1.152496337890625  ActiveDisplayYMaximum=1.239166259765625  DataLoggingVariableName=ScopeData29
      Scope2 settings: ActiveDisplayYMinimum=-1.2986907958984375  ActiveDisplayYMaximum=1.3983001708984375  DataLoggingVariableName=ScopeData33
      Scope6 settings: ActiveDisplayYMinimum=-1.5119476318359375  ActiveDisplayYMaximum=1.7752532958984375  DataLoggingVariableName=ScopeData34
      Scope7 settings: ActiveDisplayYMinimum=-0.13697814941406247  ActiveDisplayYMaximum=1.2328033447265625  DataLoggingVariableName=ScopeData36
  Scope3 : Scope  Commented=on  NumInputPorts=2
      settings: ActiveDisplayYMinimum=-1.152496337890625  ActiveDisplayYMaximum=1.239166259765625  DataLoggingVariableName=ScopeData30
  Scope4 : Scope  Commented=on  NumInputPorts=2
      settings: ActiveDisplayYMinimum=-1.3245849609375  ActiveDisplayYMaximum=1.3646240234375  DataLoggingVariableName=ScopeData31
  Scope5 : Scope  Commented=on  NumInputPorts=2
      settings: ActiveDisplayYMinimum=-1.5119476318359375  ActiveDisplayYMaximum=1.7752532958984375  DataLoggingVariableName=ScopeData32
  Shift : hdlBasic/Shift  Commented=on  shift_dir=Right  shift_bits=10  en=off  latency=0  precision=Full  arith_type="Signed  (2's comp)"  n_bits=16  bin_pt=14  quantization=Truncate  overflow=Wrap  XmcBlockStatus=1  maskContainerNames=group2  block_type=shift  block_config=sysgen:Shift_config
  Shift1 : hdlBasic/Shift  shift_dir=Right  shift_bits=10  en=off  latency=0  precision=Full  arith_type="Signed  (2's comp)"  n_bits=16  bin_pt=14  quantization=Truncate  overflow=Wrap  XmcBlockStatus=1  maskContainerNames=group2  block_type=shift  block_config=sysgen:Shift_config
  Spectrum Analyzer : SpectrumAnalyzer  WindowPosition=[672.000000,50.000000,800.000000,572.000000,]  ScopeFrameLocation=window  WindowInvariantSamplesPerUpdate=on  Span=27000  StartFrequency=-13500  StopFrequency=13500  YLimits=[-59.2094 9.1556]
  Spectrum Analyzer1 : SpectrumAnalyzer  Commented=on  WindowPosition=[396.000000,1267.000000,800.000000,500.000000,]  ScopeFrameLocation=window  WindowInvariantSamplesPerUpdate=on  Span=27000  StartFrequency=-13500  StopFrequency=13500  YLimits=[-74.9951 11.2982]
  Spectrum Analyzer2 : SpectrumAnalyzer  Commented=on  WindowPosition=[386.000000,659.000000,800.000000,500.000000,]  ScopeFrameLocation=window  WindowInvariantSamplesPerUpdate=on  Span=27000  StartFrequency=-13500  StopFrequency=13500  YLimits=[-153.5542 19.2426]
  Spectrum Analyzer3 : SpectrumAnalyzer  WindowPosition=[509.000000,561.000000,800.000000,500.000000,]  ScopeFrameLocation=window  WindowInvariantSamplesPerUpdate=on  Span=27000  StartFrequency=-13500  StopFrequency=13500  YLimits=[-67.2303 11.0236]
  SquareRoot1 : hdlBasic/SquareRoot  Commented=on  flow_control=NonBlocking  axi_optimize_goal=Resources  latency=0  rate=1  has_a_tlast=off  has_a_tuser=off  en=off  has_result_tready=off  has_invalid_op=off  fpo_op_type=square_root  has_b_tlast=false  has_b_tuser=false  result_tlast_behv=1  has_underflow=false  has_overflow=false  has_divide_by_zero=false  XmcBlockStatus=1  maskContainerNames=tabcontainer1  block_type=squareroot  block_config=sysgen:FPOBlockDescriptor_config
  SquareRoot2 : hdlBasic/SquareRoot  flow_control=NonBlocking  axi_optimize_goal=Resources  latency=0  rate=1  has_a_tlast=off  has_a_tuser=off  en=off  has_result_tready=off  has_invalid_op=off  fpo_op_type=square_root  has_b_tlast=false  has_b_tuser=false  result_tlast_behv=1  has_underflow=false  has_overflow=false  has_divide_by_zero=false  XmcBlockStatus=1  maskContainerNames=tabcontainer1  block_type=squareroot  block_config=sysgen:FPOBlockDescriptor_config
  Time Scope : Scope
      settings: TimeUnits=Metric (based on Time Span)  ActiveDisplayYMinimum=-1  ActiveDisplayYMaximum=1  YLabel=Amplitude  DataLoggingVariableName=ScopeData27
  Time Scope1 : Scope  NumInputPorts=2
      settings: TimeUnits=Metric (based on Time Span)  ActiveDisplayYMinimum=-1.068603515625  ActiveDisplayYMaximum=1.072509765625  YLabel=Amplitude  DataLoggingVariableName=ScopeData35
  Time Scope2 : Scope
      settings: TimeUnits=Metric (based on Time Span)  ActiveDisplayYMinimum=-0.17901611328125  ActiveDisplayYMaximum=0.69073486328125  YLabel=Amplitude  DataLoggingVariableName=ScopeData37
  Time Division Demultiplexer : hdlBasic/Time Division Demultiplexer  frame_pattern=[1 1 1]  impl_style=Multiple Channel  vin=off  explicit_period=off  period=1  XmcBlockStatus=1  maskContainerNames=group2  block_type=tdd  block_config=sysgen:TDD_config
  Time Division Demultiplexer1 : hdlBasic/Time Division Demultiplexer  frame_pattern=[1 1 1]  impl_style=Multiple Channel  vin=on  explicit_period=off  period=1  XmcBlockStatus=1  maskContainerNames=group2  block_type=tdd  block_config=sysgen:TDD_config
  Time Division Demultiplexer2 : hdlBasic/Time Division Demultiplexer  frame_pattern=[1 1 1]  impl_style=Multiple Channel  vin=on  explicit_period=off  period=1  XmcBlockStatus=1  maskContainerNames=group2  block_type=tdd  block_config=sysgen:TDD_config
  Time Division Demultiplexer3 : hdlBasic/Time Division Demultiplexer  frame_pattern=[1 1 1]  impl_style=Multiple Channel  vin=on  explicit_period=off  period=1  XmcBlockStatus=1  maskContainerNames=group2  block_type=tdd  block_config=sysgen:TDD_config
  Time Division Multiplexer : hdlBasic/Time Division Multiplexer  inputs=3  vin=off  Optimization=Resource  explicit_period=off  period=1  XmcBlockStatus=1  maskContainerNames=group3  block_type=tdm  block_config=sysgen:TDM_config
  To Workspace : ToWorkspace  VariableName=simout  SaveFormat=Timeseries  SampleTime=-1
  To Workspace1 : ToWorkspace  Commented=on  VariableName=complex1  SampleTime=-1
  To Workspace10 : ToWorkspace  VariableName=x1  SampleTime=-1
  To Workspace2 : ToWorkspace  Commented=on  VariableName=complex3  SampleTime=-1
  To Workspace3 : ToWorkspace  Commented=on  VariableName=complex4  SampleTime=-1
  To Workspace4 : ToWorkspace  VariableName=x  SampleTime=-1
  To Workspace5 : ToWorkspace  VariableName=x2  SampleTime=-1
  To Workspace6 : ToWorkspace  Commented=on  VariableName=complex  SampleTime=-1
  To Workspace7 : ToWorkspace  Commented=on  VariableName=complex2  SampleTime=-1
  To Workspace8 : ToWorkspace  Commented=on  VariableName=y  SampleTime=-1
  To Workspace9 : ToWorkspace  Commented=on  VariableName=z  SampleTime=-1
  Out1 : Outport
  Out2 : Outport  Port=2
  Out3 : Outport  Port=3
  Out4 : Outport  Port=4
  Out5 : Outport  Port=5
  wires:
  In1/1 -> Gateway In AXIS/1
  In2/1 -> Gateway In AXIS/2
  In3/1 -> Gateway Out AXIS/3
  Gateway In AXIS/3 -> Out3/1
  Gateway Out AXIS/2 -> Out2/1
  Gateway Out AXIS/1 -> Out1/1
  Gateway In AXIS/1 -> "FIR Compiler 7.2 "/1, Time Division Demultiplexer/1
  Time Division Demultiplexer/3 -> Gateway Out17/1, Gateway Out AXIS/1
  Time Division Demultiplexer1/3 -> Gateway Out19/1, Convert4/1, Scope5/1
  Time Division Demultiplexer1/2 -> Convert7/1, Scope4/1
  FIR Compiler 7.2 1/3 -> Time Division Demultiplexer2/1
  "FIR Compiler 7.2 "/3 -> Time Division Demultiplexer1/1, FIR Compiler 7.2 1/1
  "FIR Compiler 7.2 "/2 -> Time Division Demultiplexer1/2
  FIR Compiler 7.2 1/2 -> Time Division Demultiplexer2/2
  Time Division Demultiplexer2/2 -> Convert1/1, Scope4/2
  Time Division Demultiplexer2/3 -> Convert6/1, Scope5/2
  "FIR Compiler 7.2 "/1 -> Gateway In AXIS/3
  Gateway In AXIS/2 -> Gateway Out AXIS/2
  Time Division Demultiplexer2/1 -> Gateway Out18/1, Convert3/1, Scope3/2
  Time Division Demultiplexer1/1 -> Convert5/1, Scope3/1
  Time Division Demultiplexer2/4 -> CORDIC 6.0 2/1, CORDIC 6.0 1/1, "CORDIC 6.0 "/1
  Gateway Out5/1 -> To Workspace6/1
  Delay1/1 -> AddSub/2, AddSub1/2
  Shift/1 -> AddSub/1
  AddSub1/1 -> Shift/1
  AddSub/1 -> AddSub2/2, Delay1/1
  AddSub2/1 -> Gateway Out6/1
  Gateway Out6/1 -> To Workspace7/1
  SquareRoot1/1 -> ?
  Constant4/1 -> Relational/2
  Constant1/1 -> "Fast Fourier Transform 9.1 "/8, "Fast Fourier Transform 9.1 "/7, "Fast Fourier Transform 9.1 "/2
  Mult3/1 -> AddSub4/2
  Mult2/1 -> AddSub4/1
  Constant/1 -> "Fast Fourier Transform 9.1 "/3
  Relational/1 -> "Fast Fourier Transform 9.1 "/6
  "Fast Fourier Transform 9.1 "/5 -> Mult3/1, Mult3/2
  "Fast Fourier Transform 9.1 "/6 -> Mult2/1, Mult2/2
  Counter/1 -> Relational/1
  AddSub4/1 -> Convert2/1
  "Fast Fourier Transform 9.1 "/8 -> ?
  Convert2/1 -> SquareRoot1/1
  FIR Compiler 7.2 2/3 -> AddSub2/1, AddSub1/1
  Constant3/1 -> "Fast Fourier Transform 9.1 "/1
  Convert4/1 -> "CORDIC 6.0 "/3
  Convert3/1 -> "CORDIC 6.0 "/2
  Convert1/1 -> CORDIC 6.0 1/2
  Convert5/1 -> CORDIC 6.0 1/3
  Convert6/1 -> CORDIC 6.0 2/2
  Convert7/1 -> CORDIC 6.0 2/3
  CORDIC 6.0 1/3 -> Gateway Out1/1, Time Division Multiplexer/2
  Gateway Out1/1 -> To Workspace1/1
  CORDIC 6.0 2/3 -> Time Division Multiplexer/3, Gateway Out2/1
  Gateway Out2/1 -> To Workspace2/1
  Gateway Out3/1 -> To Workspace3/1
  Time Division Multiplexer/1 -> FIR Compiler 7.2 3/1, Gateway Out3/1
  Gateway Out7/1 -> Spectrum Analyzer/1, To Workspace4/1
  Gateway Out8/1 -> To Workspace8/1
  Gateway Out9/1 -> To Workspace9/1
  Time Division Demultiplexer3/2 -> Gateway Out8/1
  Time Division Demultiplexer3/3 -> Gateway Out9/1
  Fast Fourier Transform 9.1 1/8 -> Gateway Out10/1
  Fast Fourier Transform 9.1 1/6 -> Mult1/1, Mult1/2
  Convert8/1 -> SquareRoot2/1
  Constant2/1 -> Fast Fourier Transform 9.1 1/3
  Counter1/1 -> Relational1/1
  Relational1/1 -> Gateway Out14/1, Fast Fourier Transform 9.1 1/6
  AddSub3/1 -> Convert8/1
  Mult1/1 -> AddSub3/1
  Mult4/1 -> AddSub3/2
  Constant6/1 -> Fast Fourier Transform 9.1 1/1
  Fast Fourier Transform 9.1 1/5 -> Mult4/1, Mult4/2
  Constant5/1 -> Fast Fourier Transform 9.1 1/2, Fast Fourier Transform 9.1 1/8, Fast Fourier Transform 9.1 1/7
  SquareRoot2/1 -> Gateway Out13/1, Gateway Out/1
  Constant7/1 -> Relational1/2
  Time Division Demultiplexer3/4 -> Fast Fourier Transform 9.1 1/5
  Shift1/1 -> AddSub5/1
  AddSub5/1 -> AddSub7/2, Delay2/1
  Delay2/1 -> AddSub5/2, AddSub6/2
  AddSub6/1 -> Shift1/1
  AddSub7/1 -> Gateway Out11/1, Convert9/1
  Time Division Demultiplexer3/1 -> AddSub7/1, AddSub6/1, Gateway Out7/1
  Gateway Out/1 -> Out5/1
  Gateway Out10/1 -> Out4/1
  Convert9/1 -> Fast Fourier Transform 9.1 1/4
  Gateway Out11/1 -> Spectrum Analyzer3/1, Time Scope2/1, To Workspace10/1
  FIR Compiler 7.2 3/2 -> Time Division Demultiplexer3/2
  FIR Compiler 7.2 3/3 -> Gateway Out4/1, Time Division Demultiplexer3/1
  Gateway Out4/1 -> Spectrum Analyzer1/1
  Gateway Out12/1 -> Spectrum Analyzer2/1
  "CORDIC 6.0 "/3 -> Gateway Out12/1, Time Division Multiplexer/1, Gateway Out5/1, Gateway Out20/1, FIR Compiler 7.2 2/1
  Gateway Out13/1 -> To Workspace5/1, Time Scope/1
  Gateway Out14/1 -> Scope/1
  Time Division Demultiplexer/1 -> Gateway Out15/1
  Time Division Demultiplexer/2 -> Gateway Out16/1
  Gateway Out15/1 -> To Workspace/1, Scope1/1
  Gateway Out16/1 -> Scope2/1
  Gateway Out17/1 -> Scope6/1
  Gateway Out18/1 -> Time Scope1/1
  Gateway Out19/1 -> Time Scope1/2
  Gateway Out20/1 -> Scope7/1
